simulink model "continuousSys"  (R2020b)
settings: Solver=VariableStepAuto  StartTime=0.0  StopTime=10.0  RelTol=1e-3
settings Model: Creator=ethan  LastModifiedBy=ethan

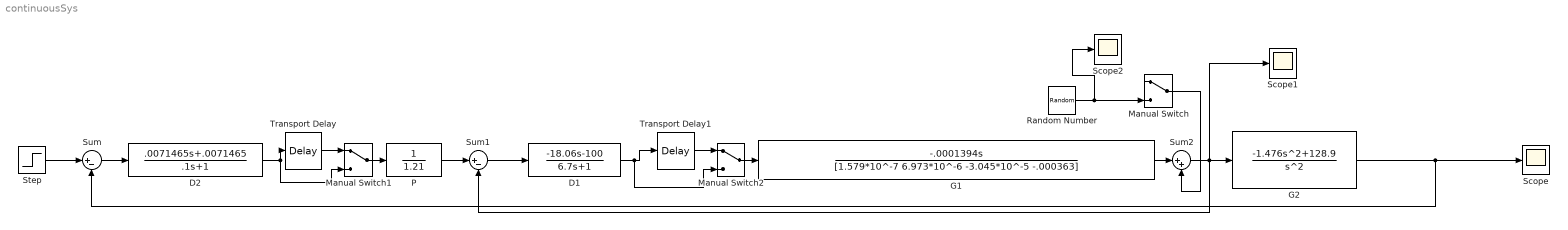
== system continuousSys ==
  D1 : TransferFcn  Numerator=[-18.06 -100]  Denominator=[6.7 1]
  D2 : TransferFcn  Numerator=[.0071465 .0071465]  Denominator=[.1 1]
  G1 : TransferFcn  Numerator=[-.0001394 0]  Denominator=[1.579*10^-7 6.973*10^-6 -3.045*10^-5 -.000363]
  G2 : TransferFcn  Numerator=[-1.476 0 128.9]  Denominator=[1 0 0]
  Manual Switch : ManualSwitch
  Manual Switch1 : ManualSwitch
  Manual Switch2 : ManualSwitch
  P : TransferFcn  Denominator=[1.21]
  Random Number : RandomNumber  Variance=.001  SampleTime=0.01
  Scope : Scope
  Scope1 : Scope
  Scope2 : Scope
  Step : Step  SampleTime=0
  Sum : Sum  Inputs=|+-
  Sum1 : Sum  Inputs=|+-
  Sum2 : Sum  Inputs=|++
  Transport Delay : TransportDelay  DelayTime=1/20
  Transport Delay1 : TransportDelay  DelayTime=1/200  PadeOrder=1
  wires:
  G2/1 -> Scope/1, Sum/2
  Sum/1 -> D2/1
  Step/1 -> Sum/1
  P/1 -> Sum1/1
  G1/1 -> Sum2/1
  Sum2/1 -> Scope1/1, Sum1/2, G2/1
  Manual Switch/1 -> Sum2/2
  Manual Switch1/1 -> P/1
  D2/1 -> Manual Switch1/2, Transport Delay/1
  Transport Delay/1 -> Manual Switch1/1
  Transport Delay1/1 -> Manual Switch2/1
  D1/1 -> Manual Switch2/2, Transport Delay1/1
  Manual Switch2/1 -> G1/1
  Sum1/1 -> D1/1
  Random Number/1 -> Scope2/1, Manual Switch/2
